simulink model "Basic_Aufbau_Explanation"  (R2013b)
settings: Solver=ode45  StartTime=0.0  StopTime=10.0  RelTol=1e-3
settings Model: Creator=daltdoer  LastModifiedBy=daltdoer

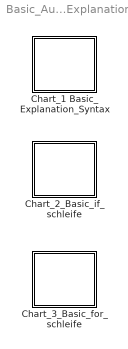
== system Basic_Aufbau_Explanation ==
  Chart_1 Basic_Explanation_Syntax : Stateflow chart  TreatAsAtomicUnit=on
  Chart_2_Basic_if_schleife : Stateflow chart  TreatAsAtomicUnit=on
  Chart_3_Basic_for_schleife : Stateflow chart  TreatAsAtomicUnit=on

== stateflow chart Basic_Aufbau_Explanation/Chart_1 Basic_Explanation_Syntax ==
  note: Default Transition:
      | legt fest, welcher Zustand nach erstmaliger Ausführung aktiv sein soll
  state Name Zustand/
    entry: Aktion 1; %wenn der Zustand aktiviert wird
    during: Aktion 2; %wenn der Zustand aktiv ist (und das Chart ausgeführt wird)
    exit: Aktion 3; %wenn der Zustand verlassen wird
    on event Aktion 4; %wenn der Zustand aktiv ist und das angegebene Ereignis auftritt
  state Name Zustand 2/
    entry: Aktion 1; %wenn der Zustand aktiviert wird
    during: Aktion 2; %wenn der Zustand aktiv ist (und das Chart ausgeführt wird)
    exit: Aktion 3; %wenn der Zustand verlassen wird
    on event Aktion 4; %wenn der Zustand aktiv ist und das angegebene Ereignis auftritt
  note: Ein Transitionslabel besitzt die Syntax:
  note: Transition ist gültig, WENN:
      | -Ausgangszustand aktiv, insofern kein Ereignis oder Bedingung angegeben
      | -das Ereignis "event" eintritt
      | -die angegebene Bedingung "condition" TRUE ist
  (default) -> Name Zustand : u
  Name Zustand -> Name Zustand 2 : event[condition==1]{conditionAction}/transitionAction

== stateflow chart Basic_Aufbau_Explanation/Chart_2_Basic_if_schleife ==
  note: Flussdiagramm mit if Abfrage
  (default) -> (junction 12)
  (junction 12) -> (junction 14) [order 1] : [a>b]
  (junction 14) -> (junction 18) [order 1] : [a>c]{aktion1}
  (junction 14) -> (junction 18) [order 2] : {aktion2}
  (junction 12) -> (junction 18) [order 2] : {aktion3;z++}

== stateflow chart Basic_Aufbau_Explanation/Chart_3_Basic_for_schleife ==
  note: Flussdiagramm for schleife
  state ?
  state ?
  (default) -> ?
  ? -> (junction 12) : E_eins{i=0}
  (junction 12) -> (junction 12) [order 1] : [i<10]
      | {i++;k=k*2}
  (junction 12) -> ? [order 2]
